simulink model "unitdelay_complex_test"  (Simulink 8.4)
settings: Solver=ode45  StartTime=0.0  StopTime=10.0  RelTol=1e-3
settings Model: Creator=arnaud  LastModifiedBy=arnaud
settings DataIOCC: SaveFormat=Structure
settings DebuggingCC: StrictBusMsg=Warning

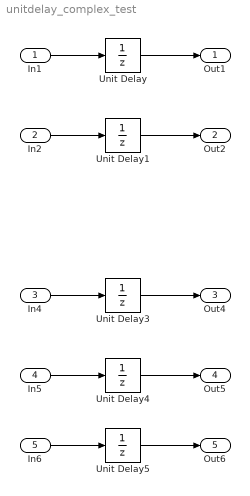
== system unitdelay_complex_test ==
  In1 : Inport  OutDataTypeStr=double  PortDimensions=1
      settings: SignalType=complex
  In2 : Inport  Port=2  OutDataTypeStr=double  PortDimensions=1
      settings: SignalType=complex
  In4 : Inport  Port=3  OutDataTypeStr=int8  PortDimensions=1
      settings: SignalType=complex
  In5 : Inport  Port=4  OutDataTypeStr=int8  PortDimensions=1
      settings: SignalType=complex
  In6 : Inport  Port=5  OutDataTypeStr=int8  PortDimensions=1
      settings: SignalType=complex
  Unit Delay : UnitDelay
  Unit Delay1 : UnitDelay  InitialCondition=0.0
  Unit Delay3 : UnitDelay
  Unit Delay4 : UnitDelay  InitialCondition=0.0
  Unit Delay5 : UnitDelay  InitialCondition=true
  Out1 : Outport
  Out2 : Outport  Port=2
  Out4 : Outport  Port=3
  Out5 : Outport  Port=4
  Out6 : Outport  Port=5
  wires:
  In1/1 -> Unit Delay/1
  Unit Delay/1 -> Out1/1
  In2/1 -> Unit Delay1/1
  Unit Delay1/1 -> Out2/1
  In4/1 -> Unit Delay3/1
  Unit Delay3/1 -> Out4/1
  In5/1 -> Unit Delay4/1
  Unit Delay4/1 -> Out5/1
  In6/1 -> Unit Delay5/1
  Unit Delay5/1 -> Out6/1
